simulink model "motor_tf"  (R2017b)
settings: Solver=ode3  StartTime=0.0  StopTime=80  FixedStep=0.1  RelTol=1e-3  EnableMultiTasking=on
libraries: simulink_need_slupdate x1
settings Model: Creator=adgp97  LastModifiedBy=adgp97

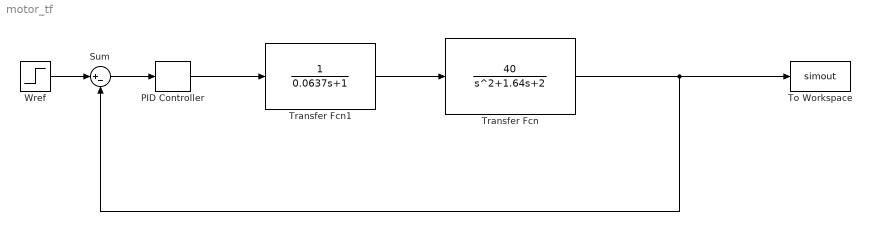
== system motor_tf ==
  PID Controller : simulink_need_slupdate/PID Controller  P=0.685  I=0  D=0
      settings: SourceProductName=Simulink
  Sum : Sum  Inputs=|+-  InputSameDT=on  OutDataTypeStr=Inherit: Same as first input
  To Workspace : ToWorkspace  VariableName=simout  SampleTime=-1
  Transfer Fcn : TransferFcn  Numerator=[40]  Denominator=[1 1.64 2]
  Transfer Fcn1 : TransferFcn  Denominator=[0.0637 1]
  Wref : Step  Time=30  Before=102  After=112
  wires:
  Transfer Fcn1/1 -> Transfer Fcn/1
  Wref/1 -> Sum/1
  Sum/1 -> PID Controller/1
  PID Controller/1 -> Transfer Fcn1/1
  Transfer Fcn/1 -> To Workspace/1, Sum/2
